simulink model "testWaterTankModel"  (R2024b)
settings: Solver=FixedStepAuto  StartTime=0.0  StopTime=10.0  RelTol=1e-3
undefined symbols (not defined in the file): InputFlowRate, OutputFlowRate, TankArea
settings Model: Creator=felipe  LastModifiedBy=felipe
settings OptimizationCC: PassReuseOutputArgsAs=Individual arguments  OptimizeBlockOrder=speed  DifferentSizesBufferReuse=on  EfficientTunableParamExpr=on
settings DebuggingCC: ParameterTunabilityLossMsg=error
settings HardwareCC: TargetBitPerLong=64  TargetBitPerPointer=64  TargetBitPerSizeT=64  TargetBitPerPtrDiffT=64  TargetLongLongMode=on  TargetIntDivRoundTo=Zero  TargetEndianess=LittleEndian  TargetWordSize=64  TargetHWDeviceType=MATLAB Host  ProdEqTarget=off
settings SFSimCC: MATLABDynamicMemAlloc=off
settings RTWCC: Description=Embedded Coder (host-based shared library target)  SystemTargetFile=ert_shrlib.tlc  TemplateMakefile=ert_default_tmf  RTWVerbose=off
settings RTWCC: CustomSourceCode=|
  | #define CONCAT(str1, str2, str3) CONCAT_(str1, str2, str3)
  | #define CONCAT_(str1, str2, str3) str1 ## str2 ## str3
  | #define GET_MMI_FUNC    CONCAT(MODEL     , _GetCAPImmi ,    )
  | #define RT_MODEL_STRUCT CONCAT(RT_MODEL_ , MODEL       , _T )
  | 
  | void* GET_MMI_FUNC(void* voidPtrToRealTimeStructure)
  | {
  |    rtwCAPI_ModelMappingInfo* mmiPtr = &(rtmGetDataMapInfo( ( RT_MODEL_STRUCT * )(voidPtrToRealTimeStructure) ).mmi);
  |    return (void*) mmiPtr;
  | }
settings CodeAppCC: GenerateComments=off  IgnoreCustomStorageClasses=off  OperatorAnnotations=on  SimulinkDataObjDesc=on  SFDataObjDesc=on  SimulinkBlockComments=off
settings STFCustomTargetCC: TargetLangStandard=C99 (ISO)  MultiwordLength=256  ParMdlRefBuildCompliant=on  CompOptLevelCompliant=on  IncludeMdlTerminateFcn=off  CombineOutputUpdateFcns=on  CombineSignalStateStructs=on  SuppressErrorStatus=on  ERTCustomFileBanners=on  SupportAbsoluteTime=off  CodeInterfacePackaging=Reusable function  SupportComplex=off  SupportContinuousTime=off  SupportNonInlinedSFcns=off  RemoveResetFunc=on  MATLABClassNameForMDSCustomization=Simulink.SoftwareTarget.ERTCustomization  ModelStepFunctionPrototypeControlCompliant=on  GenerateAllocFcn=on  UseToolchainInfoCompliant=on  SystemTargetFile=ert_shrlib.tlc
settings ERTTargetCC: TargetLangStandard=C99 (ISO)  ConcurrentExecutionCompliant=off  IncludeMdlTerminateFcn=off  CombineSignalStateStructs=on  SuppressErrorStatus=on  SupportAbsoluteTime=off  CodeInterfacePackaging=Reusable function  SupportComplex=off  CPPClassGenCompliant=off  GenerateAllocFcn=on  InlinedParameterPlacement=Hierarchical  RootIOFormat=Part of model data structure  RTWCAPIParams=on  RTWCAPIRootIO=on  ERTCustomFileTemplate=example_file_process.tlc

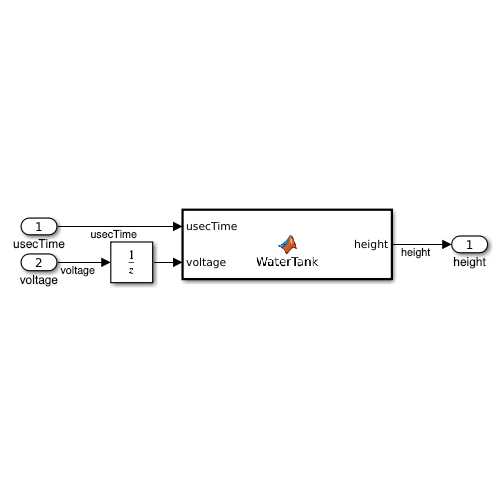
[thumbnail: Simulink's stored preview of the top-level diagram]
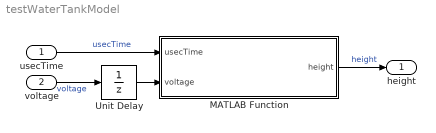
== system testWaterTankModel ==
  usecTime : Inport
  voltage : Inport  Port=2
  MATLAB Function : MATLAB Function  TreatAsAtomicUnit=on
  Unit Delay : UnitDelay  SampleTime=-1  HasFrameUpgradeWarning=on
  height : Outport
  wires:
  voltage/1 -> Unit Delay/1  "voltage"
  usecTime/1 -> MATLAB Function/1(usecTime)  "usecTime"
  MATLAB Function/1(height) -> height/1  "height"
  Unit Delay/1 -> MATLAB Function/2(voltage)

== matlab function testWaterTankModel/MATLAB Function ==
  data: usecTime input; height output; voltage input size=1; InputFlowRate parameter; OutputFlowRate parameter; TankArea parameter
function height = WaterTank(usecTime, voltage, InputFlowRate, OutputFlowRate, TankArea)

% Persistent variables - these maintain their values after every call of
% the function
persistent lastHeight lastUsecTime
if isempty(lastHeight)
    % Initialization
    voltage = 0;
    lastHeight = 0;
    lastUsecTime = 0;
end

% Simple Euler method
height = (voltage * OutputFlowRate - InputFlowRate * sqrt(lastHeight)) / TankArea * (usecTime - lastUsecTime) + lastHeight;

    if height < 0
        warning('WaterTank: Height is negative, setting to 0');
        height = 0;
    end

%  Update the last state
lastHeight = height;
lastUsecTime = usecTime;

end
